simulink model "Intergration_ACC"  (R2018b)
settings: Solver=FixedStepDiscrete  StartTime=0.0  StopTime=inf  FixedStep=0.005  RelTol=1e-3
PostLoadFcn:
  | if any(exist('dsrtsu_mdlpostloadfcn', 'file') ~= 0), dsrtsu_mdlpostloadfcn('Execute', bdroot); end
values from neighbouring files (symbols this model uses):
  P_x165_On = 1.0    [CAN_Tx.sldd]
  P_x242_On = 1.0    [CAN_Tx.sldd]
  P_x246_On = 1.0    [CAN_Tx.sldd]
libraries: rtican x112, simulink x59
(part 31 of 31)

== system Intergration_ACC/TX/RADAR_HSC2_FrP01_0x244/Subsystem9 ==
  AEBPedtrnSysFltSts : Inport
  AEBAlvRlngCtr : Inport  Port=2
  Add : Sum
  Bitwise Operator1 : simulink/Logic and Bit Operations/Bitwise Operator  logicop=AND  UseBitMask=on  BitMask=bin2dec('00001111')  BitMaskRealWorld=Stored Integer
  Bitwise Operator3 : simulink/Logic and Bit Operations/Bitwise Operator  logicop=AND  UseBitMask=on  BitMask=bin2dec('01110000')  BitMaskRealWorld=Stored Integer
  Data Type Conversion1 : DataTypeConversion  OutDataTypeStr=uint8
  Data Type Conversion3 : DataTypeConversion  OutDataTypeStr=uint8
  Shift Arithmetic2 : ArithShift  BitShiftNumber=4  BitShiftDirection=Left
  x244_byte4 : Outport
  wires:
  Bitwise Operator1/1 -> Add/2
  Bitwise Operator3/1 -> Add/1
  Data Type Conversion1/1 -> Bitwise Operator1/1
  AEBAlvRlngCtr/1 -> Data Type Conversion1/1
  AEBPedtrnSysFltSts/1 -> Data Type Conversion3/1
  Shift Arithmetic2/1 -> Bitwise Operator3/1
  Add/1 -> x244_byte4/1
  Data Type Conversion3/1 -> Shift Arithmetic2/1

== system Intergration_ACC/TX/YRS1_0x131/RollingCounter1 ==
  Add2 : Sum
  Constant5 : Constant
  Constant6 : Constant  Value=-1
  Delay : Delay  DelayLength=1
  Switch : Switch  Criteria=u2 > Threshold  Threshold=14
  RC : Outport
  wires:
  Constant6/1 -> Switch/1
  Switch/1 -> Add2/2
  Delay/1 -> RC/1, Switch/3, Switch/2
  Add2/1 -> Delay/1
  Constant5/1 -> Add2/1

== system Intergration_ACC/TX/YRS1_0x131/Subsystem ==
  In1 : Inport
  Add : Sum
  Add1 : Sum  Inputs=+-
  Bitwise Operator1 : simulink/Logic and Bit Operations/Bitwise Operator  logicop=AND  UseBitMask=on  BitMask=bin2dec('11111111')  BitMaskRealWorld=Stored Integer
  Bitwise Operator2 : simulink/Logic and Bit Operations/Bitwise Operator  logicop=AND  UseBitMask=on  BitMask=bin2dec('11111111')  BitMaskRealWorld=Stored Integer
  Constant1 : Constant  Value=2
  Constant2 : Constant  Value=0.001
  Constant3 : Constant  Value=0.001
  Constant4 : Constant  Value=2
  Data Type Conversion1 : DataTypeConversion  OutDataTypeStr=uint16
  Data Type Conversion2 : DataTypeConversion  OutDataTypeStr=uint8
  Data Type Conversion3 : DataTypeConversion  OutDataTypeStr=uint8
  Divide1 : Product  Inputs=*/
  Multiply : Product
  Shift Arithmetic1 : ArithShift  BitShiftNumber=8  BitShiftDirection=Right
  Byte2 : Outport
  Out2 : Outport  Port=2
  Byte3 : Outport  Port=3
  wires:
  Constant2/1 -> Divide1/2
  Constant1/1 -> Add/2
  Data Type Conversion1/1 -> Bitwise Operator2/1, Multiply/1, Shift Arithmetic1/1
  Shift Arithmetic1/1 -> Bitwise Operator1/1
  Constant4/1 -> Add1/2
  Constant3/1 -> Multiply/2
  Multiply/1 -> Add1/1
  Bitwise Operator1/1 -> Data Type Conversion2/1
  Divide1/1 -> Data Type Conversion1/1
  Add/1 -> Divide1/1
  Add1/1 -> Out2/1
  Bitwise Operator2/1 -> Data Type Conversion3/1
  In1/1 -> Add/1
  Data Type Conversion2/1 -> Byte2/1
  Data Type Conversion3/1 -> Byte3/1

== system Intergration_ACC/TX/YRS1_0x131/Subsystem1 ==
  In1 : Inport
  Add : Sum
  Add1 : Sum  Inputs=+-
  Bitwise Operator1 : simulink/Logic and Bit Operations/Bitwise Operator  logicop=AND  UseBitMask=on  BitMask=bin2dec('11111111')  BitMaskRealWorld=Stored Integer
  Bitwise Operator2 : simulink/Logic and Bit Operations/Bitwise Operator  logicop=AND  UseBitMask=on  BitMask=bin2dec('11111111')  BitMaskRealWorld=Stored Integer
  Constant1 : Constant  Value=180
  Constant2 : Constant  Value=0.01
  Constant3 : Constant  Value=0.01
  Constant4 : Constant  Value=180
  Data Type Conversion1 : DataTypeConversion  OutDataTypeStr=uint16
  Data Type Conversion2 : DataTypeConversion  OutDataTypeStr=uint8
  Data Type Conversion3 : DataTypeConversion  OutDataTypeStr=uint8
  Divide1 : Product  Inputs=*/
  Multiply : Product
  Shift Arithmetic1 : ArithShift  BitShiftNumber=8  BitShiftDirection=Right
  Byte4 : Outport
  Out2 : Outport  Port=2
  Byte5 : Outport  Port=3
  wires:
  Constant2/1 -> Divide1/2
  Constant1/1 -> Add/2
  Data Type Conversion1/1 -> Bitwise Operator2/1, Multiply/1, Shift Arithmetic1/1
  Shift Arithmetic1/1 -> Bitwise Operator1/1
  Constant4/1 -> Add1/2
  Constant3/1 -> Multiply/2
  Multiply/1 -> Add1/1
  Bitwise Operator1/1 -> Data Type Conversion3/1
  Divide1/1 -> Data Type Conversion1/1
  Add/1 -> Divide1/1
  Add1/1 -> Out2/1
  Bitwise Operator2/1 -> Data Type Conversion2/1
  In1/1 -> Add/1
  Data Type Conversion2/1 -> Byte5/1
  Data Type Conversion3/1 -> Byte4/1

== system Intergration_ACC/TX/YRS1_0x131/Subsystem4 ==
  In1 : Inport
  Bitwise Operator2 : simulink/Logic and Bit Operations/Bitwise Operator  logicop=AND  UseBitMask=on  BitMask=bin2dec('00001111')  BitMaskRealWorld=Stored Integer
  Data Type Conversion1 : DataTypeConversion  OutDataTypeStr=uint8
  Byte6 : Outport
  wires:
  In1/1 -> Data Type Conversion1/1
  Bitwise Operator2/1 -> Byte6/1
  Data Type Conversion1/1 -> Bitwise Operator2/1

== system Intergration_ACC/TX/YRS2_0x132/RollingCounter1 ==
  Add2 : Sum
  Constant5 : Constant
  Constant6 : Constant  Value=-1
  Delay : Delay  DelayLength=1
  Switch : Switch  Criteria=u2 > Threshold  Threshold=14
  RC : Outport
  wires:
  Constant6/1 -> Switch/1
  Switch/1 -> Add2/2
  Delay/1 -> RC/1, Switch/3, Switch/2
  Add2/1 -> Delay/1
  Constant5/1 -> Add2/1

== system Intergration_ACC/TX/YRS2_0x132/Subsystem ==
  In1 : Inport
  Add : Sum
  Add1 : Sum  Inputs=+-
  Bitwise Operator1 : simulink/Logic and Bit Operations/Bitwise Operator  logicop=AND  UseBitMask=on  BitMask=bin2dec('11111111')  BitMaskRealWorld=Stored Integer
  Bitwise Operator2 : simulink/Logic and Bit Operations/Bitwise Operator  logicop=AND  UseBitMask=on  BitMask=bin2dec('11111111')  BitMaskRealWorld=Stored Integer
  Constant1 : Constant  Value=2
  Constant2 : Constant  Value=0.001
  Constant3 : Constant  Value=0.001
  Constant4 : Constant  Value=2
  Data Type Conversion1 : DataTypeConversion  OutDataTypeStr=uint16
  Data Type Conversion2 : DataTypeConversion  OutDataTypeStr=uint8
  Data Type Conversion3 : DataTypeConversion  OutDataTypeStr=uint8
  Divide1 : Product  Inputs=*/
  Multiply : Product
  Shift Arithmetic1 : ArithShift  BitShiftNumber=8  BitShiftDirection=Right
  Byte2 : Outport
  Out2 : Outport  Port=2
  Byte3 : Outport  Port=3
  wires:
  Constant2/1 -> Divide1/2
  Constant1/1 -> Add/2
  Data Type Conversion1/1 -> Bitwise Operator2/1, Multiply/1, Shift Arithmetic1/1
  Shift Arithmetic1/1 -> Bitwise Operator1/1
  Constant4/1 -> Add1/2
  Constant3/1 -> Multiply/2
  Multiply/1 -> Add1/1
  Bitwise Operator1/1 -> Data Type Conversion2/1
  Divide1/1 -> Data Type Conversion1/1
  Add/1 -> Divide1/1
  Add1/1 -> Out2/1
  Bitwise Operator2/1 -> Data Type Conversion3/1
  In1/1 -> Add/1
  Data Type Conversion2/1 -> Byte2/1
  Data Type Conversion3/1 -> Byte3/1

== system Intergration_ACC/TX/YRS2_0x132/Subsystem4 ==
  In1 : Inport
  Bitwise Operator2 : simulink/Logic and Bit Operations/Bitwise Operator  logicop=AND  UseBitMask=on  BitMask=bin2dec('00001111')  BitMaskRealWorld=Stored Integer
  Data Type Conversion1 : DataTypeConversion  OutDataTypeStr=uint8
  Byte6 : Outport
  wires:
  In1/1 -> Data Type Conversion1/1
  Bitwise Operator2/1 -> Byte6/1
  Data Type Conversion1/1 -> Bitwise Operator2/1

== system Intergration_ACC/RTI Data/RTI Data Store/RTI Data Store/RTI Data Store ==
  RTI Data Store : Subsystem  mask(RTI_DATA_STORE){}
      mask help:
      | RTI Data Store Block. This block is used by RTI to store internal model dependent data. Deleting this block will result in data loss.
      |
      | NEVER DELETE, COPY, OR MODIFY THIS BLOCK!
      mask Help:
      | RTI Data Store Block. This block is used by RTI to store internal model dependent data. Deleting this block will result in data loss.
      | 
      | NEVER DELETE, COPY, OR MODIFY THIS BLOCK!
      mask Display: text(0.5, 0.5, ' ', 'HorizontalAlignment', 'center');

== system Intergration_ACC/RTI Data/RTI Data Store/RTI Data Store/RTI Data Store/RTI Data Store ==

== stateflow chart Intergration_ACC/OutputSignal_OS ==
  settings: description=_0p0.DUMMY.222_000_
  (default) -> (junction 68)
  (junction 68) -> (junction 67) : {
      | i= i+1;
      | }
  (junction 67) -> (junction 63) [order 1] : [ i%%2== 0]
  (junction 67) -> (junction 62) [order 2]
  (junction 63) -> (junction 61) : {
      | do_10ms;
      | }
  (junction 61) -> (junction 62)
  (junction 62) -> (junction 87)
  (junction 87) -> (junction 88) [order 1] : [ i%%4==0]
  (junction 87) -> (junction 89) [order 2]
  (junction 88) -> (junction 90) : {
      | do_20ms;
      | }
  (junction 90) -> (junction 89)
  (junction 89) -> (junction 108)
  (junction 108) -> (junction 107) [order 1] : [ i>=200]
  (junction 108) -> (junction 109) [order 2]
  (junction 107) -> (junction 110) : {
      | i=0;
      | }
  (junction 110) -> (junction 109)
  data: i local int32
  events: do_20ms output FUNCTION_CALL_EVENT; do_10ms output FUNCTION_CALL_EVENT
